simulink model "secuencia"  (R2016a)
settings: Solver=VariableStepAuto  StartTime=0.0  StopTime=10.0  RelTol=1e-3
values from neighbouring files (symbols this model uses):
  bitsInfo = [0 0 1]    [matrizGeneradora.m]
  tb = 0.06    [matrizGeneradora.m]
libraries: simulink_extras x4, simulink x2, commrandsrc3 x1
settings Model: Creator=Leandro  LastModifiedBy=leand

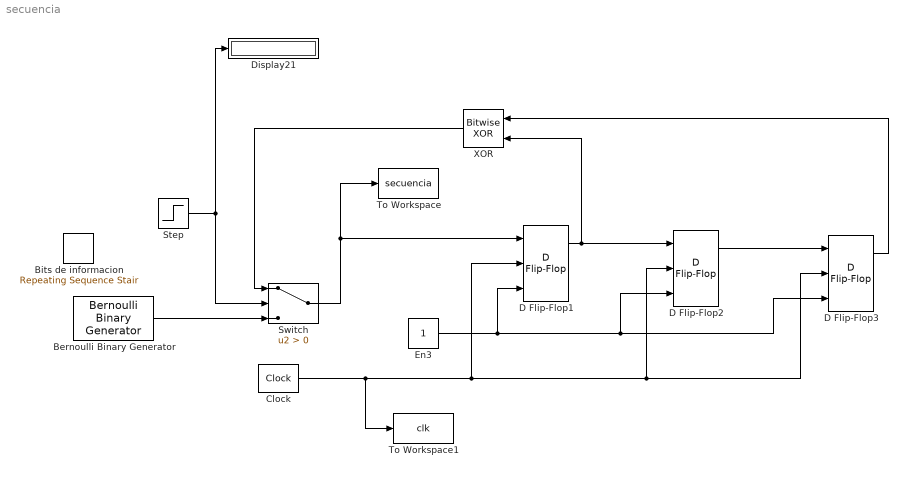
== system secuencia ==
  Bernoulli Binary Generator : commrandsrc3/Bernoulli Binary Generator  ProbabilityOfZero=0.5  SeedSource=Auto  Seed=0  SampleTime=1  SamplesPerFrame=1  OutputDataType=double  SimulateUsing=Interpreted execution
  Bits de informacion : simulink/Sources/Repeating Sequence Stair  OutValues=[0 bitsInfo zeros(1,30) ]'  tsamp=tb  OutMin=[]  OutMax=[]  OutDataTypeStr=fixdt('boolean')  OutputDataTypeScalingMode=Specify via dialog  OutDataType=fixdt('boolean')  ConRadixGroup=Best Precision: Vector-wise  OutScaling=[]
  Clock : simulink_extras/Flip Flops/Clock  period=tb
  D Flip-Flop1 : simulink_extras/Flip Flops/D Flip-Flop
  D Flip-Flop2 : simulink_extras/Flip Flops/D Flip-Flop
  D Flip-Flop3 : simulink_extras/Flip Flops/D Flip-Flop
  Display21 : Display
  En3 : Constant
  Step : Step  SampleTime=6.5*tb
  Switch : Switch  Criteria=u2 > Threshold
  To Workspace : ToWorkspace  VariableName=secuencia  SaveFormat=Timeseries  SampleTime=-1
  To Workspace1 : ToWorkspace  VariableName=clk  SaveFormat=Timeseries  SampleTime=-1
  "XOR " : simulink/Logic and Bit Operations/Bitwise Operator  logicop=XOR  UseBitMask=off  NumInputPorts=2  BitMask=bin2dec('11011001')  BitMaskRealWorld=Stored Integer
  wires:
  Switch/1 -> D Flip-Flop1/1, To Workspace/1
  En3/1 -> D Flip-Flop1/3, D Flip-Flop2/3, D Flip-Flop3/3
  Clock/1 -> To Workspace1/1, D Flip-Flop1/2, D Flip-Flop2/2, D Flip-Flop3/2
  D Flip-Flop2/1 -> D Flip-Flop3/1
  D Flip-Flop3/1 -> "XOR "/1
  D Flip-Flop1/1 -> "XOR "/2, D Flip-Flop2/1
  "XOR "/1 -> Switch/1
  Step/1 -> Switch/2, Display21/1
  Bernoulli Binary Generator/1 -> Switch/3
